simulink model "question6"  (R2022a)
settings: Solver=VariableStepAuto  StartTime=0.0  StopTime=T  RelTol=1e-3
values from neighbouring files (symbols this model uses):
  D = [0 0]'    [hw.m]
  K = lqr(A, B, Qr, Rr)    [hw.m]
  x0 = [1 0 1 0 0]'    [hw.m]
undefined symbols (not defined in the file or in its folder): A, B
settings Model: Creator=antonio  LastModifiedBy=antonio

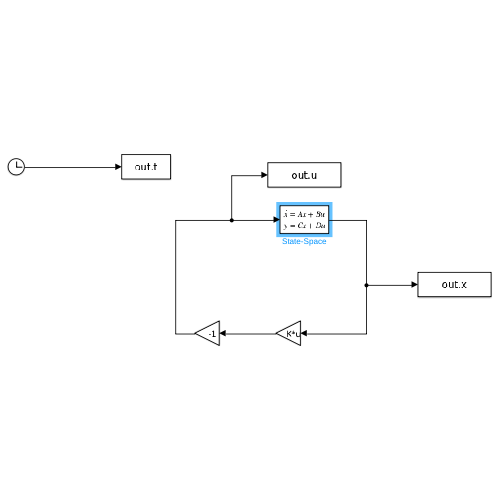
[thumbnail: Simulink's stored preview of the top-level diagram]
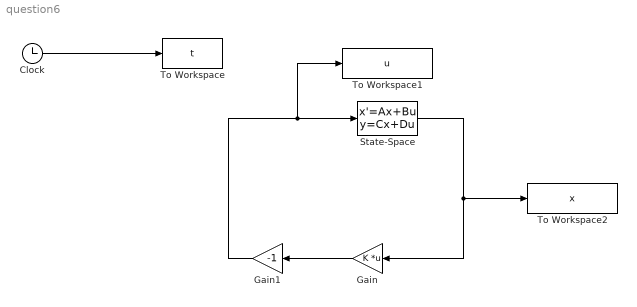
== system question6 ==
  Clock : Clock
  Gain : Gain  Gain=K  Multiplication=Matrix(K*u)
  Gain1 : Gain  Gain=-1
  State-Space : StateSpace  A=A  B=B  C=eye(5)  D=D  InitialCondition=x0  ContinuousStateAttributes='State'
  To Workspace : ToWorkspace  VariableName=t  SampleTime=-1
  To Workspace1 : ToWorkspace  VariableName=u  SampleTime=-1
  To Workspace2 : ToWorkspace  VariableName=x  SampleTime=-1
  wires:
  Clock/1 -> To Workspace/1
  State-Space/1 -> Gain/1, To Workspace2/1
  Gain/1 -> Gain1/1
  Gain1/1 -> To Workspace1/1, State-Space/1
